simulink model "attitude3d"  (R2019b)
settings: Solver=ode4  StartTime=0.0  StopTime=6530  FixedStep=10  RelTol=1e-3
values from neighbouring files (symbols this model uses):
  antenna_vb = [1, 0, 0]    [attitude3d_init.m]
  init_xBI = [1, 0, 0]    [attitude3d_init.m]
  init_yBI = [0, 1, 0]    [attitude3d_init.m]
  init_zBI = [0, 0, 1]    [attitude3d_init.m]
  P = 2 * pi / mean_motion    [attitude3d_init.m]
  solar_array_vb = [1, 0, 0]    [attitude3d_init.m]
  star_sensor_1_vb = [1/sqrt(2), +1/sqrt(2), 0]    [attitude3d_init.m]
  star_sensor_2_vb = [1/sqrt(2), -1/sqrt(2), 0]    [attitude3d_init.m]
  target_mean_radius = mean_mars_radius    (= 3389500)    [attitude3d_init.m]
  thrust_no_shadow_weight = 1.0    (= 1)    [attitude3d_init.m]
  thrust_shadow_weight = 1.0    (= 1)    [attitude3d_init.m]
  thruster_vb = [-1, 0, 0]    [attitude3d_init.m]
  window_n = int16(window_t/10.0)    [attitude3d_init.m]
  x = [0,        max_omega*0.1,  0, 0               ;      0.5 * P,  max_omega*0.1,  0, 0               ;      1.0 * P,  max_omega*0.1,  0, 0               ]    [attitude3d_init.m]
libraries: vrlib x14, simulink x6, dspstat3 x4, commfilt2 x2
(part 2 of 2)

== system attitude3d/frame change4/transposeQuaternion ==
  q : Inport
  Gain1 : Gain  Gain=[1 -1 -1 -1]  SaturateOnIntegerOverflow=on  OutDataTypeStr=Inherit: Same as input  ParamDataTypeStr=Inherit: Same as input
  q' : Outport
  wires:
  q/1 -> Gain1/1
  Gain1/1 -> q'/1

== system attitude3d/quat2rot/Norm ==
  X : Inport
  Dot Product1 : DotProduct  InputSameDT=on  OutDataTypeStr=Inherit: Inherit via internal rule
  Math Function : Math  Operator=sqrt  SaturateOnIntegerOverflow=on
  ||X|| : Outport  InitialOutput=0
  wires:
  Math Function/1 -> ||X||/1
  Dot Product1/1 -> Math Function/1
  X/1 -> Dot Product1/2, Dot Product1/1

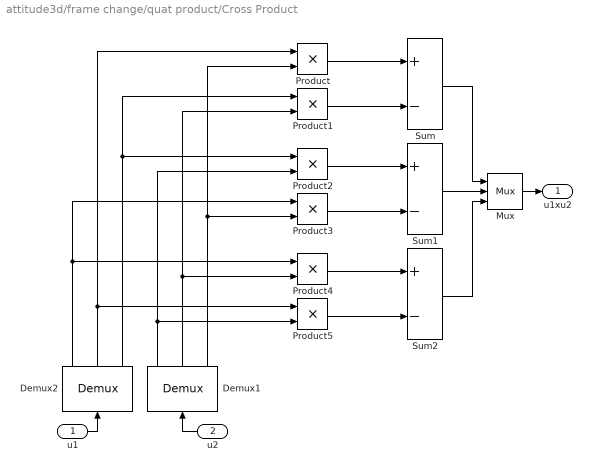
== system attitude3d/frame change/quat product/Cross Product ==
  u1 : Inport
  u2 : Inport  Port=2
  Demux1 : Demux  Outputs=3
  Demux2 : Demux  Outputs=3
  Mux : Mux  Inputs=3
  Product{,1..5} (6 alike) : Product  SaturateOnIntegerOverflow=on  RndMeth=Zero  InputSameDT=on  OutDataTypeStr=Inherit: Same as first input
  Sum : Sum  Inputs=+-  SaturateOnIntegerOverflow=on  InputSameDT=on  OutDataTypeStr=Inherit: Same as first input
  Sum1 : Sum  Inputs=+-  SaturateOnIntegerOverflow=on  InputSameDT=on  OutDataTypeStr=Inherit: Same as first input
  Sum2 : Sum  Inputs=+-  SaturateOnIntegerOverflow=on  InputSameDT=on  OutDataTypeStr=Inherit: Same as first input
  u1xu2 : Outport  InitialOutput=0
  wires:
  u2/1 -> Demux1/1
  u1/1 -> Demux2/1
  Mux/1 -> u1xu2/1
  Product/1 -> Sum/1
  Product1/1 -> Sum/2
  Product2/1 -> Sum1/1
  Product3/1 -> Sum1/2
  Product4/1 -> Sum2/1
  Product5/1 -> Sum2/2
  Demux2/3 -> Product1/1, Product2/1
  Demux1/3 -> Product/2, Product3/2
  Demux2/1 -> Product3/1, Product4/1
  Demux1/2 -> Product1/2, Product4/2
  Demux2/2 -> Product/1, Product5/1
  Demux1/1 -> Product2/2, Product5/2
  Sum/1 -> Mux/1
  Sum1/1 -> Mux/2
  Sum2/1 -> Mux/3

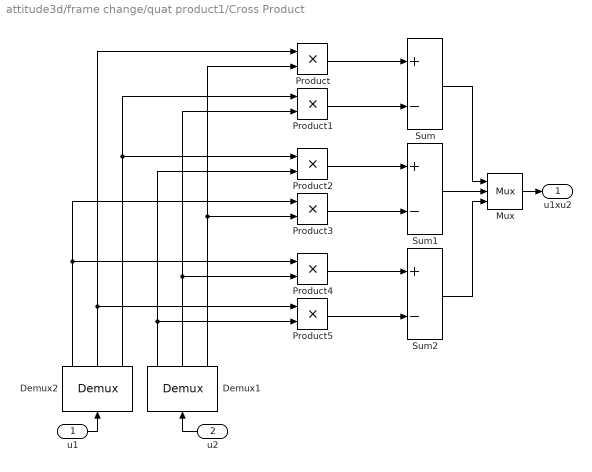
== system attitude3d/frame change/quat product1/Cross Product ==
  u1 : Inport
  u2 : Inport  Port=2
  Demux1 : Demux  Outputs=3
  Demux2 : Demux  Outputs=3
  Mux : Mux  Inputs=3
  Product{,1..5} (6 alike) : Product  SaturateOnIntegerOverflow=on  RndMeth=Zero  InputSameDT=on  OutDataTypeStr=Inherit: Same as first input
  Sum : Sum  Inputs=+-  SaturateOnIntegerOverflow=on  InputSameDT=on  OutDataTypeStr=Inherit: Same as first input
  Sum1 : Sum  Inputs=+-  SaturateOnIntegerOverflow=on  InputSameDT=on  OutDataTypeStr=Inherit: Same as first input
  Sum2 : Sum  Inputs=+-  SaturateOnIntegerOverflow=on  InputSameDT=on  OutDataTypeStr=Inherit: Same as first input
  u1xu2 : Outport  InitialOutput=0
  wires:
  Sum2/1 -> Mux/3
  Sum1/1 -> Mux/2
  Sum/1 -> Mux/1
  Demux1/1 -> Product5/2, Product2/2
  Demux2/2 -> Product5/1, Product/1
  Demux1/2 -> Product4/2, Product1/2
  Demux2/1 -> Product4/1, Product3/1
  Demux1/3 -> Product3/2, Product/2
  Demux2/3 -> Product2/1, Product1/1
  Product5/1 -> Sum2/2
  Product4/1 -> Sum2/1
  Product3/1 -> Sum1/2
  Product2/1 -> Sum1/1
  Product1/1 -> Sum/2
  Product/1 -> Sum/1
  Mux/1 -> u1xu2/1
  u1/1 -> Demux2/1
  u2/1 -> Demux1/1

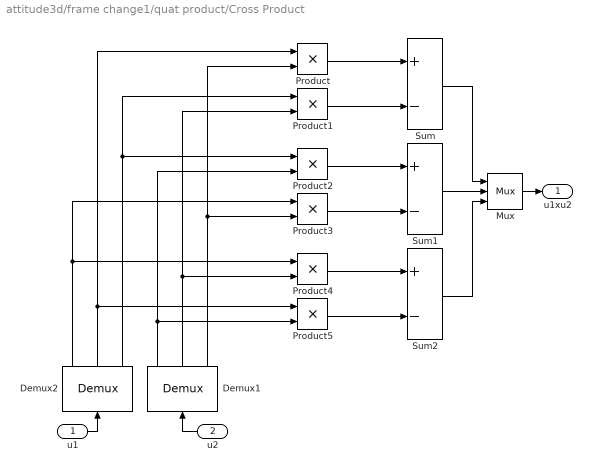
== system attitude3d/frame change1/quat product/Cross Product ==
  u1 : Inport
  u2 : Inport  Port=2
  Demux1 : Demux  Outputs=3
  Demux2 : Demux  Outputs=3
  Mux : Mux  Inputs=3
  Product{,1..5} (6 alike) : Product  SaturateOnIntegerOverflow=on  RndMeth=Zero  InputSameDT=on  OutDataTypeStr=Inherit: Same as first input
  Sum : Sum  Inputs=+-  SaturateOnIntegerOverflow=on  InputSameDT=on  OutDataTypeStr=Inherit: Same as first input
  Sum1 : Sum  Inputs=+-  SaturateOnIntegerOverflow=on  InputSameDT=on  OutDataTypeStr=Inherit: Same as first input
  Sum2 : Sum  Inputs=+-  SaturateOnIntegerOverflow=on  InputSameDT=on  OutDataTypeStr=Inherit: Same as first input
  u1xu2 : Outport  InitialOutput=0
  wires:
  u2/1 -> Demux1/1
  u1/1 -> Demux2/1
  Mux/1 -> u1xu2/1
  Product/1 -> Sum/1
  Product1/1 -> Sum/2
  Product2/1 -> Sum1/1
  Product3/1 -> Sum1/2
  Product4/1 -> Sum2/1
  Product5/1 -> Sum2/2
  Demux2/3 -> Product1/1, Product2/1
  Demux1/3 -> Product/2, Product3/2
  Demux2/1 -> Product3/1, Product4/1
  Demux1/2 -> Product1/2, Product4/2
  Demux2/2 -> Product/1, Product5/1
  Demux1/1 -> Product2/2, Product5/2
  Sum/1 -> Mux/1
  Sum1/1 -> Mux/2
  Sum2/1 -> Mux/3

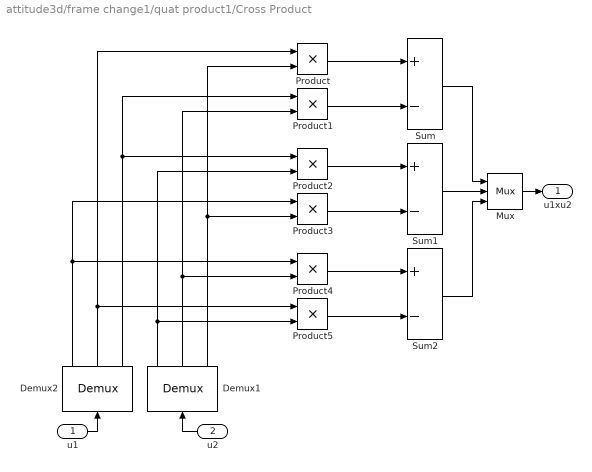
== system attitude3d/frame change1/quat product1/Cross Product ==
  u1 : Inport
  u2 : Inport  Port=2
  Demux1 : Demux  Outputs=3
  Demux2 : Demux  Outputs=3
  Mux : Mux  Inputs=3
  Product{,1..5} (6 alike) : Product  SaturateOnIntegerOverflow=on  RndMeth=Zero  InputSameDT=on  OutDataTypeStr=Inherit: Same as first input
  Sum : Sum  Inputs=+-  SaturateOnIntegerOverflow=on  InputSameDT=on  OutDataTypeStr=Inherit: Same as first input
  Sum1 : Sum  Inputs=+-  SaturateOnIntegerOverflow=on  InputSameDT=on  OutDataTypeStr=Inherit: Same as first input
  Sum2 : Sum  Inputs=+-  SaturateOnIntegerOverflow=on  InputSameDT=on  OutDataTypeStr=Inherit: Same as first input
  u1xu2 : Outport  InitialOutput=0
  wires:
  Sum2/1 -> Mux/3
  Sum1/1 -> Mux/2
  Sum/1 -> Mux/1
  Demux1/1 -> Product5/2, Product2/2
  Demux2/2 -> Product5/1, Product/1
  Demux1/2 -> Product4/2, Product1/2
  Demux2/1 -> Product4/1, Product3/1
  Demux1/3 -> Product3/2, Product/2
  Demux2/3 -> Product2/1, Product1/1
  Product5/1 -> Sum2/2
  Product4/1 -> Sum2/1
  Product3/1 -> Sum1/2
  Product2/1 -> Sum1/1
  Product1/1 -> Sum/2
  Product/1 -> Sum/1
  Mux/1 -> u1xu2/1
  u1/1 -> Demux2/1
  u2/1 -> Demux1/1

== system attitude3d/frame change2/quat product/Cross Product ==
  u1 : Inport
  u2 : Inport  Port=2
  Demux1 : Demux  Outputs=3
  Demux2 : Demux  Outputs=3
  Mux : Mux  Inputs=3
  Product{,1..5} (6 alike) : Product  SaturateOnIntegerOverflow=on  RndMeth=Zero  InputSameDT=on  OutDataTypeStr=Inherit: Same as first input
  Sum : Sum  Inputs=+-  SaturateOnIntegerOverflow=on  InputSameDT=on  OutDataTypeStr=Inherit: Same as first input
  Sum1 : Sum  Inputs=+-  SaturateOnIntegerOverflow=on  InputSameDT=on  OutDataTypeStr=Inherit: Same as first input
  Sum2 : Sum  Inputs=+-  SaturateOnIntegerOverflow=on  InputSameDT=on  OutDataTypeStr=Inherit: Same as first input
  u1xu2 : Outport  InitialOutput=0
  wires:
  u2/1 -> Demux1/1
  u1/1 -> Demux2/1
  Mux/1 -> u1xu2/1
  Product/1 -> Sum/1
  Product1/1 -> Sum/2
  Product2/1 -> Sum1/1
  Product3/1 -> Sum1/2
  Product4/1 -> Sum2/1
  Product5/1 -> Sum2/2
  Demux2/3 -> Product1/1, Product2/1
  Demux1/3 -> Product/2, Product3/2
  Demux2/1 -> Product3/1, Product4/1
  Demux1/2 -> Product1/2, Product4/2
  Demux2/2 -> Product/1, Product5/1
  Demux1/1 -> Product2/2, Product5/2
  Sum/1 -> Mux/1
  Sum1/1 -> Mux/2
  Sum2/1 -> Mux/3

== system attitude3d/frame change2/quat product1/Cross Product ==
  u1 : Inport
  u2 : Inport  Port=2
  Demux1 : Demux  Outputs=3
  Demux2 : Demux  Outputs=3
  Mux : Mux  Inputs=3
  Product{,1..5} (6 alike) : Product  SaturateOnIntegerOverflow=on  RndMeth=Zero  InputSameDT=on  OutDataTypeStr=Inherit: Same as first input
  Sum : Sum  Inputs=+-  SaturateOnIntegerOverflow=on  InputSameDT=on  OutDataTypeStr=Inherit: Same as first input
  Sum1 : Sum  Inputs=+-  SaturateOnIntegerOverflow=on  InputSameDT=on  OutDataTypeStr=Inherit: Same as first input
  Sum2 : Sum  Inputs=+-  SaturateOnIntegerOverflow=on  InputSameDT=on  OutDataTypeStr=Inherit: Same as first input
  u1xu2 : Outport  InitialOutput=0
  wires:
  Sum2/1 -> Mux/3
  Sum1/1 -> Mux/2
  Sum/1 -> Mux/1
  Demux1/1 -> Product5/2, Product2/2
  Demux2/2 -> Product5/1, Product/1
  Demux1/2 -> Product4/2, Product1/2
  Demux2/1 -> Product4/1, Product3/1
  Demux1/3 -> Product3/2, Product/2
  Demux2/3 -> Product2/1, Product1/1
  Product5/1 -> Sum2/2
  Product4/1 -> Sum2/1
  Product3/1 -> Sum1/2
  Product2/1 -> Sum1/1
  Product1/1 -> Sum/2
  Product/1 -> Sum/1
  Mux/1 -> u1xu2/1
  u1/1 -> Demux2/1
  u2/1 -> Demux1/1

== system attitude3d/frame change3/quat product/Cross Product ==
  u1 : Inport
  u2 : Inport  Port=2
  Demux1 : Demux  Outputs=3
  Demux2 : Demux  Outputs=3
  Mux : Mux  Inputs=3
  Product{,1..5} (6 alike) : Product  SaturateOnIntegerOverflow=on  RndMeth=Zero  InputSameDT=on  OutDataTypeStr=Inherit: Same as first input
  Sum : Sum  Inputs=+-  SaturateOnIntegerOverflow=on  InputSameDT=on  OutDataTypeStr=Inherit: Same as first input
  Sum1 : Sum  Inputs=+-  SaturateOnIntegerOverflow=on  InputSameDT=on  OutDataTypeStr=Inherit: Same as first input
  Sum2 : Sum  Inputs=+-  SaturateOnIntegerOverflow=on  InputSameDT=on  OutDataTypeStr=Inherit: Same as first input
  u1xu2 : Outport  InitialOutput=0
  wires:
  u2/1 -> Demux1/1
  u1/1 -> Demux2/1
  Mux/1 -> u1xu2/1
  Product/1 -> Sum/1
  Product1/1 -> Sum/2
  Product2/1 -> Sum1/1
  Product3/1 -> Sum1/2
  Product4/1 -> Sum2/1
  Product5/1 -> Sum2/2
  Demux2/3 -> Product1/1, Product2/1
  Demux1/3 -> Product/2, Product3/2
  Demux2/1 -> Product3/1, Product4/1
  Demux1/2 -> Product1/2, Product4/2
  Demux2/2 -> Product/1, Product5/1
  Demux1/1 -> Product2/2, Product5/2
  Sum/1 -> Mux/1
  Sum1/1 -> Mux/2
  Sum2/1 -> Mux/3

== system attitude3d/frame change3/quat product1/Cross Product ==
  u1 : Inport
  u2 : Inport  Port=2
  Demux1 : Demux  Outputs=3
  Demux2 : Demux  Outputs=3
  Mux : Mux  Inputs=3
  Product{,1..5} (6 alike) : Product  SaturateOnIntegerOverflow=on  RndMeth=Zero  InputSameDT=on  OutDataTypeStr=Inherit: Same as first input
  Sum : Sum  Inputs=+-  SaturateOnIntegerOverflow=on  InputSameDT=on  OutDataTypeStr=Inherit: Same as first input
  Sum1 : Sum  Inputs=+-  SaturateOnIntegerOverflow=on  InputSameDT=on  OutDataTypeStr=Inherit: Same as first input
  Sum2 : Sum  Inputs=+-  SaturateOnIntegerOverflow=on  InputSameDT=on  OutDataTypeStr=Inherit: Same as first input
  u1xu2 : Outport  InitialOutput=0
  wires:
  Sum2/1 -> Mux/3
  Sum1/1 -> Mux/2
  Sum/1 -> Mux/1
  Demux1/1 -> Product5/2, Product2/2
  Demux2/2 -> Product5/1, Product/1
  Demux1/2 -> Product4/2, Product1/2
  Demux2/1 -> Product4/1, Product3/1
  Demux1/3 -> Product3/2, Product/2
  Demux2/3 -> Product2/1, Product1/1
  Product5/1 -> Sum2/2
  Product4/1 -> Sum2/1
  Product3/1 -> Sum1/2
  Product2/1 -> Sum1/1
  Product1/1 -> Sum/2
  Product/1 -> Sum/1
  Mux/1 -> u1xu2/1
  u1/1 -> Demux2/1
  u2/1 -> Demux1/1

== system attitude3d/frame change4/quat product/Cross Product ==
  u1 : Inport
  u2 : Inport  Port=2
  Demux1 : Demux  Outputs=3
  Demux2 : Demux  Outputs=3
  Mux : Mux  Inputs=3
  Product{,1..5} (6 alike) : Product  SaturateOnIntegerOverflow=on  RndMeth=Zero  InputSameDT=on  OutDataTypeStr=Inherit: Same as first input
  Sum : Sum  Inputs=+-  SaturateOnIntegerOverflow=on  InputSameDT=on  OutDataTypeStr=Inherit: Same as first input
  Sum1 : Sum  Inputs=+-  SaturateOnIntegerOverflow=on  InputSameDT=on  OutDataTypeStr=Inherit: Same as first input
  Sum2 : Sum  Inputs=+-  SaturateOnIntegerOverflow=on  InputSameDT=on  OutDataTypeStr=Inherit: Same as first input
  u1xu2 : Outport  InitialOutput=0
  wires:
  u2/1 -> Demux1/1
  u1/1 -> Demux2/1
  Mux/1 -> u1xu2/1
  Product/1 -> Sum/1
  Product1/1 -> Sum/2
  Product2/1 -> Sum1/1
  Product3/1 -> Sum1/2
  Product4/1 -> Sum2/1
  Product5/1 -> Sum2/2
  Demux2/3 -> Product1/1, Product2/1
  Demux1/3 -> Product/2, Product3/2
  Demux2/1 -> Product3/1, Product4/1
  Demux1/2 -> Product1/2, Product4/2
  Demux2/2 -> Product/1, Product5/1
  Demux1/1 -> Product2/2, Product5/2
  Sum/1 -> Mux/1
  Sum1/1 -> Mux/2
  Sum2/1 -> Mux/3

== system attitude3d/frame change4/quat product1/Cross Product ==
  u1 : Inport
  u2 : Inport  Port=2
  Demux1 : Demux  Outputs=3
  Demux2 : Demux  Outputs=3
  Mux : Mux  Inputs=3
  Product{,1..5} (6 alike) : Product  SaturateOnIntegerOverflow=on  RndMeth=Zero  InputSameDT=on  OutDataTypeStr=Inherit: Same as first input
  Sum : Sum  Inputs=+-  SaturateOnIntegerOverflow=on  InputSameDT=on  OutDataTypeStr=Inherit: Same as first input
  Sum1 : Sum  Inputs=+-  SaturateOnIntegerOverflow=on  InputSameDT=on  OutDataTypeStr=Inherit: Same as first input
  Sum2 : Sum  Inputs=+-  SaturateOnIntegerOverflow=on  InputSameDT=on  OutDataTypeStr=Inherit: Same as first input
  u1xu2 : Outport  InitialOutput=0
  wires:
  Sum2/1 -> Mux/3
  Sum1/1 -> Mux/2
  Sum/1 -> Mux/1
  Demux1/1 -> Product5/2, Product2/2
  Demux2/2 -> Product5/1, Product/1
  Demux1/2 -> Product4/2, Product1/2
  Demux2/1 -> Product4/1, Product3/1
  Demux1/3 -> Product3/2, Product/2
  Demux2/3 -> Product2/1, Product1/1
  Product5/1 -> Sum2/2
  Product4/1 -> Sum2/1
  Product3/1 -> Sum1/2
  Product2/1 -> Sum1/1
  Product1/1 -> Sum/2
  Product/1 -> Sum/1
  Mux/1 -> u1xu2/1
  u1/1 -> Demux2/1
  u2/1 -> Demux1/1

== matlab function attitude3d/frame2quat1/MATLAB Function ==
  data: xB input; qA2B output; yB input; zB input
function qA2B = frame2quat(xB,yB,zB)
%#codegen

A = zeros(1,4);
T = [xB(:),yB(:),zB(:)];
qA2B = zeros(4,1);

A(1) =  T(1,1) + T(2,2) + T(3,3);
A(2) =  T(1,1) - T(2,2) - T(3,3);
A(3) = -T(1,1) + T(2,2) - T(3,3);
A(4) = -T(1,1) - T(2,2) + T(3,3);

[~,idx] = max(A);

switch idx
    case 1
        qA2B(1) = 0.5*sqrt(1+A(1));
        D = 1/(4*qA2B(1));
        qA2B(2) = (T(3,2)-T(2,3))*D;
        qA2B(3) = (T(1,3)-T(3,1))*D;
        qA2B(4) = (T(2,1)-T(1,2))*D;
    case 2
        qA2B(2) = 0.5*sqrt(1+A(2));
        D = 1/(4*qA2B(2));
        qA2B(3) = (T(2,1)+T(1,2))*D;
        qA2B(4) = (T(1,3)+T(3,1))*D;
        qA2B(1) = (T(3,2)-T(2,3))*D;
    case 3
        qA2B(3) = 0.5*sqrt(1+A(3));
        D = 1/(4*qA2B(3));
        qA2B(4) = (T(3,2)+T(2,3))*D;
        qA2B(1) = (T(1,3)-T(3,1))*D;
        qA2B(2) = (T(2,1)+T(1,2))*D;
    case 4
        qA2B(4) = 0.5*sqrt(1+A(4));
        D = 1/(4*qA2B(4));
        qA2B(1) = (T(2,1)-T(1,2))*D;
        qA2B(2) = (T(1,3)+T(3,1))*D;
        qA2B(3) = (T(3,2)+T(2,3))*D;
end % switch

== matlab function attitude3d/Interpolator  ==
  data: x input; omega output; t input
function omega = interp(x, t)
t_p =   x(:,1);
o_p_x = x(:,2);
o_p_y = x(:,3);
o_p_z = x(:,4);
omega = [interp1(t_p, o_p_x, t); ...
         interp1(t_p, o_p_y, t); ...
         interp1(t_p, o_p_z, t)];

== matlab function attitude3d/Quaternion Propagator/Quaternion Differential ==
  data: q input; q_dot output; omega input
function q_dot = q_diff(q, omega)
q_dot = 0.5 * [0        , -omega(1), -omega(2), -omega(1);
                omega(3),         0,  omega(1), -omega(2);
                omega(2), -omega(1), 0        , -omega(3);
               omega(1), omega(2), -omega(3),        0] * [q(1);
                                                           q(2);
                                                           q(3);
                                                           q(4)];

== matlab function attitude3d/Quaternion Propagator/Quaternion Normed ==
  data: u input; y output
function y = quatnorm(u)


y = u/ norm(u);
